simulink model "DCE_motor6_V2"  (R2025a)
settings: Solver=ode4  StartTime=0.0  StopTime=1  FixedStep=5e-5  RelTol=1e-3
undefined symbols (not defined in the file or in its folder): powergui
libraries: spsControlledVoltageSourceLib x24, spsControlledCurrentSourceLib x24, spsVoltageMeasurementLib x24, slpidlib x24, spspowerguiLib x2, simulink x1
(part 4 of 5)

== system DCE_motor6_V2/joint4/Motor2 ==
  TL : Inport
  IR_in : Inport  Port=2
  L_in : Inport  Port=3
  psi_in : Inport  Port=4
  2 : Gain  Gain=4
  Connector : Subsystem
  Constant : Constant  Value=-pi/2
  Constant1 : Constant  Value=2*pi
  Constant2 : Constant  Value=2*pi
  Gain : Gain  Gain=-50
  Integrator : Integrator
  Mechanical : Subsystem
  Mod : Math  Operator=mod
  Mod1 : Math  Operator=mod
  Mod2 : Math  Operator=mod
  Mux : Mux  Inputs=2
  P : Gain  Gain=50
  Product{,1..2,4} (4 alike) : Product
  Product3 : Product  Inputs=*/
  Sin : Trigonometry
  Sin1 : Trigonometry
  Sin2 : Trigonometry
  Sum : Sum  Inputs=+--
  Sum of Elements : Sum  Inputs=+
  Sum1 : Sum
  Sum2 : Sum
  Td : Gain  Gain=-0.003
  A+ : PMIOPort  Side=Left
  A- : PMIOPort  Port=2  Side=Left
  B+ : PMIOPort  Port=3  Side=Left
  B- : PMIOPort  Port=4  Side=Left
  Vp : Outport
  Ip : Outport  Port=2
  Te : Outport  Port=3
  w : Outport  Port=4
  theta : Outport  Port=5
  wires:
  Sum/1 -> Product3/1
  P/1 -> Mod1/1, 2/1, Sum2/1
  Mechanical/2(theta) -> theta/1, P/1
  Mechanical/1(w) -> Product1/2, w/1
  Product/1 -> Sum of Elements/1
  Sin2/1 -> Td/1
  Td/1 -> Sum1/2
  Sin1/1 -> Mux/1
  Integrator/1 -> Product2/1, Product/1, Ip/1, Connector/1(Ip)
  Constant/1 -> Sum2/2
  Sum of Elements/1 -> Sum1/1
  Connector/1(Vp) -> Vp/1, Sum/1
  Mux/1 -> Product4/1
  Sin/1 -> Mux/2
  Product1/1 -> Sum/2
  Sum1/1 -> Te/1, Mechanical/2(Te)
  TL/1 -> Mechanical/1(TL)
  Mod1/1 -> Sin1/1
  Mod/1 -> Sin/1
  Sum2/1 -> Mod/1
  Constant2/1 -> Mod/2
  Constant1/1 -> Mod1/2, Mod2/2
  Mod2/1 -> Sin2/1
  2/1 -> Mod2/1
  Product2/1 -> Sum/3
  IR_in/1 -> Product2/2
  Product3/1 -> Integrator/1
  L_in/1 -> Product3/2
  Product4/1 -> Product/2, Product1/1
  psi_in/1 -> Gain/1
  Gain/1 -> Product4/2
  connections:
  Connector/LConn4 -- B-/RConn1
  Connector/LConn3 -- B+/RConn1
  Connector/LConn2 -- A-/RConn1
  Connector/LConn1 -- A+/RConn1

== system DCE_motor6_V2/joint5/Mini08-1 ==
  In2 : Inport
  w : Inport  Port=2
  角度增益 : Gain  Gain=1/50
  转速增益 : Gain  Gain=1/50
  "Theta " : Outport
  "w " : Outport  Port=2
  wires:
  In2/1 -> 角度增益/1
  角度增益/1 -> "Theta "/1
  转速增益/1 -> "w "/1
  w/1 -> 转速增益/1

== system DCE_motor6_V2/joint5/Mini08-2 ==
  In2 : Inport
  w : Inport  Port=2
  角度增益 : Gain  Gain=1/50
  转速增益 : Gain  Gain=1/50
  "Theta " : Outport
  "w " : Outport  Port=2
  wires:
  In2/1 -> 角度增益/1
  角度增益/1 -> "Theta "/1
  转速增益/1 -> "w "/1
  w/1 -> 转速增益/1

== system DCE_motor6_V2/joint5/More Info2 ==

== system DCE_motor6_V2/joint5/Motor1 ==
  TL : Inport
  IR_in : Inport  Port=2
  L_in : Inport  Port=3
  psi_in : Inport  Port=4
  2 : Gain  Gain=4
  Connector : Subsystem
  Constant : Constant  Value=-pi/2
  Constant1 : Constant  Value=2*pi
  Constant2 : Constant  Value=2*pi
  Gain : Gain  Gain=-50
  Integrator : Integrator
  Mechanical : Subsystem
  Mod : Math  Operator=mod
  Mod1 : Math  Operator=mod
  Mod2 : Math  Operator=mod
  Mux : Mux  Inputs=2
  P : Gain  Gain=50
  Product{,1..2,4} (4 alike) : Product
  Product3 : Product  Inputs=*/
  Sin : Trigonometry
  Sin1 : Trigonometry
  Sin2 : Trigonometry
  Sum : Sum  Inputs=+--
  Sum of Elements : Sum  Inputs=+
  Sum1 : Sum
  Sum2 : Sum
  Td : Gain  Gain=-0.003
  A+ : PMIOPort  Side=Left
  A- : PMIOPort  Port=2  Side=Left
  B+ : PMIOPort  Port=3  Side=Left
  B- : PMIOPort  Port=4  Side=Left
  Vp : Outport
  Ip : Outport  Port=2
  Te : Outport  Port=3
  w : Outport  Port=4
  theta : Outport  Port=5
  wires:
  Sum/1 -> Product3/1
  P/1 -> Mod1/1, 2/1, Sum2/1
  Mechanical/2(theta) -> theta/1, P/1
  Mechanical/1(w) -> Product1/2, w/1
  Product/1 -> Sum of Elements/1
  Sin2/1 -> Td/1
  Td/1 -> Sum1/2
  Sin1/1 -> Mux/1
  Integrator/1 -> Product2/1, Product/1, Ip/1, Connector/1(Ip)
  Constant/1 -> Sum2/2
  Sum of Elements/1 -> Sum1/1
  Connector/1(Vp) -> Vp/1, Sum/1
  Mux/1 -> Product4/1
  Sin/1 -> Mux/2
  Product1/1 -> Sum/2
  Sum1/1 -> Te/1, Mechanical/2(Te)
  TL/1 -> Mechanical/1(TL)
  Mod1/1 -> Sin1/1
  Mod/1 -> Sin/1
  Sum2/1 -> Mod/1
  Constant2/1 -> Mod/2
  Constant1/1 -> Mod1/2, Mod2/2
  Mod2/1 -> Sin2/1
  2/1 -> Mod2/1
  Product2/1 -> Sum/3
  IR_in/1 -> Product2/2
  Product3/1 -> Integrator/1
  L_in/1 -> Product3/2
  Product4/1 -> Product/2, Product1/1
  psi_in/1 -> Gain/1
  Gain/1 -> Product4/2
  connections:
  Connector/LConn4 -- B-/RConn1
  Connector/LConn3 -- B+/RConn1
  Connector/LConn2 -- A-/RConn1
  Connector/LConn1 -- A+/RConn1

== system DCE_motor6_V2/joint5/Motor2 ==
  TL : Inport
  IR_in : Inport  Port=2
  L_in : Inport  Port=3
  psi_in : Inport  Port=4
  2 : Gain  Gain=4
  Connector : Subsystem
  Constant : Constant  Value=-pi/2
  Constant1 : Constant  Value=2*pi
  Constant2 : Constant  Value=2*pi
  Gain : Gain  Gain=-50
  Integrator : Integrator
  Mechanical : Subsystem
  Mod : Math  Operator=mod
  Mod1 : Math  Operator=mod
  Mod2 : Math  Operator=mod
  Mux : Mux  Inputs=2
  P : Gain  Gain=50
  Product{,1..2,4} (4 alike) : Product
  Product3 : Product  Inputs=*/
  Sin : Trigonometry
  Sin1 : Trigonometry
  Sin2 : Trigonometry
  Sum : Sum  Inputs=+--
  Sum of Elements : Sum  Inputs=+
  Sum1 : Sum
  Sum2 : Sum
  Td : Gain  Gain=-0.003
  A+ : PMIOPort  Side=Left
  A- : PMIOPort  Port=2  Side=Left
  B+ : PMIOPort  Port=3  Side=Left
  B- : PMIOPort  Port=4  Side=Left
  Vp : Outport
  Ip : Outport  Port=2
  Te : Outport  Port=3
  w : Outport  Port=4
  theta : Outport  Port=5
  wires:
  Sum/1 -> Product3/1
  P/1 -> Mod1/1, 2/1, Sum2/1
  Mechanical/2(theta) -> theta/1, P/1
  Mechanical/1(w) -> Product1/2, w/1
  Product/1 -> Sum of Elements/1
  Sin2/1 -> Td/1
  Td/1 -> Sum1/2
  Sin1/1 -> Mux/1
  Integrator/1 -> Product2/1, Product/1, Ip/1, Connector/1(Ip)
  Constant/1 -> Sum2/2
  Sum of Elements/1 -> Sum1/1
  Connector/1(Vp) -> Vp/1, Sum/1
  Mux/1 -> Product4/1
  Sin/1 -> Mux/2
  Product1/1 -> Sum/2
  Sum1/1 -> Te/1, Mechanical/2(Te)
  TL/1 -> Mechanical/1(TL)
  Mod1/1 -> Sin1/1
  Mod/1 -> Sin/1
  Sum2/1 -> Mod/1
  Constant2/1 -> Mod/2
  Constant1/1 -> Mod1/2, Mod2/2
  Mod2/1 -> Sin2/1
  2/1 -> Mod2/1
  Product2/1 -> Sum/3
  IR_in/1 -> Product2/2
  Product3/1 -> Integrator/1
  L_in/1 -> Product3/2
  Product4/1 -> Product/2, Product1/1
  psi_in/1 -> Gain/1
  Gain/1 -> Product4/2
  connections:
  Connector/LConn4 -- B-/RConn1
  Connector/LConn3 -- B+/RConn1
  Connector/LConn2 -- A-/RConn1
  Connector/LConn1 -- A+/RConn1

== system DCE_motor6_V2/joint6/Mini08-1 ==
  In2 : Inport
  w : Inport  Port=2
  角度增益 : Gain  Gain=1/50
  转速增益 : Gain  Gain=1/50
  "Theta " : Outport
  "w " : Outport  Port=2
  wires:
  In2/1 -> 角度增益/1
  角度增益/1 -> "Theta "/1
  转速增益/1 -> "w "/1
  w/1 -> 转速增益/1

== system DCE_motor6_V2/joint6/Mini08-2 ==
  In2 : Inport
  w : Inport  Port=2
  角度增益 : Gain  Gain=1/50
  转速增益 : Gain  Gain=1/50
  "Theta " : Outport
  "w " : Outport  Port=2
  wires:
  In2/1 -> 角度增益/1
  角度增益/1 -> "Theta "/1
  转速增益/1 -> "w "/1
  w/1 -> 转速增益/1

== system DCE_motor6_V2/joint6/Motor1 ==
  TL : Inport
  IR_in : Inport  Port=2
  L_in : Inport  Port=3
  psi_in : Inport  Port=4
  2 : Gain  Gain=4
  Connector : Subsystem
  Constant : Constant  Value=-pi/2
  Constant1 : Constant  Value=2*pi
  Constant2 : Constant  Value=2*pi
  Gain : Gain  Gain=-50
  Integrator : Integrator
  Mechanical : Subsystem
  Mod : Math  Operator=mod
  Mod1 : Math  Operator=mod
  Mod2 : Math  Operator=mod
  Mux : Mux  Inputs=2
  P : Gain  Gain=50
  Product{,1..2,4} (4 alike) : Product
  Product3 : Product  Inputs=*/
  Sin : Trigonometry
  Sin1 : Trigonometry
  Sin2 : Trigonometry
  Sum : Sum  Inputs=+--
  Sum of Elements : Sum  Inputs=+
  Sum1 : Sum
  Sum2 : Sum
  Td : Gain  Gain=-0.003
  A+ : PMIOPort  Side=Left
  A- : PMIOPort  Port=2  Side=Left
  B+ : PMIOPort  Port=3  Side=Left
  B- : PMIOPort  Port=4  Side=Left
  Vp : Outport
  Ip : Outport  Port=2
  Te : Outport  Port=3
  w : Outport  Port=4
  theta : Outport  Port=5
  wires:
  Sum/1 -> Product3/1
  P/1 -> Mod1/1, 2/1, Sum2/1
  Mechanical/2(theta) -> theta/1, P/1
  Mechanical/1(w) -> Product1/2, w/1
  Product/1 -> Sum of Elements/1
  Sin2/1 -> Td/1
  Td/1 -> Sum1/2
  Sin1/1 -> Mux/1
  Integrator/1 -> Product2/1, Product/1, Ip/1, Connector/1(Ip)
  Constant/1 -> Sum2/2
  Sum of Elements/1 -> Sum1/1
  Connector/1(Vp) -> Vp/1, Sum/1
  Mux/1 -> Product4/1
  Sin/1 -> Mux/2
  Product1/1 -> Sum/2
  Sum1/1 -> Te/1, Mechanical/2(Te)
  TL/1 -> Mechanical/1(TL)
  Mod1/1 -> Sin1/1
  Mod/1 -> Sin/1
  Sum2/1 -> Mod/1
  Constant2/1 -> Mod/2
  Constant1/1 -> Mod1/2, Mod2/2
  Mod2/1 -> Sin2/1
  2/1 -> Mod2/1
  Product2/1 -> Sum/3
  IR_in/1 -> Product2/2
  Product3/1 -> Integrator/1
  L_in/1 -> Product3/2
  Product4/1 -> Product/2, Product1/1
  psi_in/1 -> Gain/1
  Gain/1 -> Product4/2
  connections:
  Connector/LConn4 -- B-/RConn1
  Connector/LConn3 -- B+/RConn1
  Connector/LConn2 -- A-/RConn1
  Connector/LConn1 -- A+/RConn1

== system DCE_motor6_V2/joint6/Motor2 ==
  TL : Inport
  IR_in : Inport  Port=2
  L_in : Inport  Port=3
  psi_in : Inport  Port=4
  2 : Gain  Gain=4
  Connector : Subsystem
  Constant : Constant  Value=-pi/2
  Constant1 : Constant  Value=2*pi
  Constant2 : Constant  Value=2*pi
  Gain : Gain  Gain=-50
  Integrator : Integrator
  Mechanical : Subsystem
  Mod : Math  Operator=mod
  Mod1 : Math  Operator=mod
  Mod2 : Math  Operator=mod
  Mux : Mux  Inputs=2
  P : Gain  Gain=50
  Product{,1..2,4} (4 alike) : Product
  Product3 : Product  Inputs=*/
  Sin : Trigonometry
  Sin1 : Trigonometry
  Sin2 : Trigonometry
  Sum : Sum  Inputs=+--
  Sum of Elements : Sum  Inputs=+
  Sum1 : Sum
  Sum2 : Sum
  Td : Gain  Gain=-0.003
  A+ : PMIOPort  Side=Left
  A- : PMIOPort  Port=2  Side=Left
  B+ : PMIOPort  Port=3  Side=Left
  B- : PMIOPort  Port=4  Side=Left
  Vp : Outport
  Ip : Outport  Port=2
  Te : Outport  Port=3
  w : Outport  Port=4
  theta : Outport  Port=5
  wires:
  Sum/1 -> Product3/1
  P/1 -> Mod1/1, 2/1, Sum2/1
  Mechanical/2(theta) -> theta/1, P/1
  Mechanical/1(w) -> Product1/2, w/1
  Product/1 -> Sum of Elements/1
  Sin2/1 -> Td/1
  Td/1 -> Sum1/2
  Sin1/1 -> Mux/1
  Integrator/1 -> Product2/1, Product/1, Ip/1, Connector/1(Ip)
  Constant/1 -> Sum2/2
  Sum of Elements/1 -> Sum1/1
  Connector/1(Vp) -> Vp/1, Sum/1
  Mux/1 -> Product4/1
  Sin/1 -> Mux/2
  Product1/1 -> Sum/2
  Sum1/1 -> Te/1, Mechanical/2(Te)
  TL/1 -> Mechanical/1(TL)
  Mod1/1 -> Sin1/1
  Mod/1 -> Sin/1
  Sum2/1 -> Mod/1
  Constant2/1 -> Mod/2
  Constant1/1 -> Mod1/2, Mod2/2
  Mod2/1 -> Sin2/1
  2/1 -> Mod2/1
  Product2/1 -> Sum/3
  IR_in/1 -> Product2/2
  Product3/1 -> Integrator/1
  L_in/1 -> Product3/2
  Product4/1 -> Product/2, Product1/1
  psi_in/1 -> Gain/1
  Gain/1 -> Product4/2
  connections:
  Connector/LConn4 -- B-/RConn1
  Connector/LConn3 -- B+/RConn1
  Connector/LConn2 -- A-/RConn1
  Connector/LConn1 -- A+/RConn1

== system DCE_motor6_V2/powergui1/EquivalentModel1 ==
  Sources : Subsystem
  State-Space : S-Function  FunctionName=sfun_spssw_discc  Parameters=S.Ts,S.A, S.B, S.C, S.D, S.x0,S.EnableUseOfTLC  SFunctionDeploymentMode=off  EnableBusSupport=off
  Yout : Subsystem
  wires:
  State-Space/1 -> Yout/1(v,i)
  Sources/1(u) -> State-Space/1

== system DCE_motor6_V2/powergui1/EquivalentModel10 ==
  Sources : Subsystem
  State-Space : S-Function  FunctionName=sfun_spssw_discc  Parameters=S.Ts,S.A, S.B, S.C, S.D, S.x0,S.EnableUseOfTLC  SFunctionDeploymentMode=off  EnableBusSupport=off
  Yout : Subsystem
  wires:
  State-Space/1 -> Yout/1(v,i)
  Sources/1(u) -> State-Space/1

== system DCE_motor6_V2/powergui1/EquivalentModel11 ==
  Sources : Subsystem
  State-Space : S-Function  FunctionName=sfun_spssw_discc  Parameters=S.Ts,S.A, S.B, S.C, S.D, S.x0,S.EnableUseOfTLC  SFunctionDeploymentMode=off  EnableBusSupport=off
  Yout : Subsystem
  wires:
  State-Space/1 -> Yout/1(v,i)
  Sources/1(u) -> State-Space/1

== system DCE_motor6_V2/powergui1/EquivalentModel12 ==
  Sources : Subsystem
  State-Space : S-Function  FunctionName=sfun_spssw_discc  Parameters=S.Ts,S.A, S.B, S.C, S.D, S.x0,S.EnableUseOfTLC  SFunctionDeploymentMode=off  EnableBusSupport=off
  Yout : Subsystem
  wires:
  State-Space/1 -> Yout/1(v,i)
  Sources/1(u) -> State-Space/1

== system DCE_motor6_V2/powergui1/EquivalentModel13 ==
  Sources : Subsystem
  State-Space : S-Function  FunctionName=sfun_spssw_discc  Parameters=S.Ts,S.A, S.B, S.C, S.D, S.x0,S.EnableUseOfTLC  SFunctionDeploymentMode=off  EnableBusSupport=off
  Yout : Subsystem
  wires:
  State-Space/1 -> Yout/1(v,i)
  Sources/1(u) -> State-Space/1

== system DCE_motor6_V2/powergui1/EquivalentModel14 ==
  Sources : Subsystem
  State-Space : S-Function  FunctionName=sfun_spssw_discc  Parameters=S.Ts,S.A, S.B, S.C, S.D, S.x0,S.EnableUseOfTLC  SFunctionDeploymentMode=off  EnableBusSupport=off
  Yout : Subsystem
  wires:
  State-Space/1 -> Yout/1(v,i)
  Sources/1(u) -> State-Space/1

== system DCE_motor6_V2/powergui1/EquivalentModel15 ==
  Sources : Subsystem
  State-Space : S-Function  FunctionName=sfun_spssw_discc  Parameters=S.Ts,S.A, S.B, S.C, S.D, S.x0,S.EnableUseOfTLC  SFunctionDeploymentMode=off  EnableBusSupport=off
  Yout : Subsystem
  wires:
  State-Space/1 -> Yout/1(v,i)
  Sources/1(u) -> State-Space/1

== system DCE_motor6_V2/powergui1/EquivalentModel16 ==
  Sources : Subsystem
  State-Space : S-Function  FunctionName=sfun_spssw_discc  Parameters=S.Ts,S.A, S.B, S.C, S.D, S.x0,S.EnableUseOfTLC  SFunctionDeploymentMode=off  EnableBusSupport=off
  Yout : Subsystem
  wires:
  State-Space/1 -> Yout/1(v,i)
  Sources/1(u) -> State-Space/1

== system DCE_motor6_V2/powergui1/EquivalentModel17 ==
  Sources : Subsystem
  State-Space : S-Function  FunctionName=sfun_spssw_discc  Parameters=S.Ts,S.A, S.B, S.C, S.D, S.x0,S.EnableUseOfTLC  SFunctionDeploymentMode=off  EnableBusSupport=off
  Yout : Subsystem
  wires:
  State-Space/1 -> Yout/1(v,i)
  Sources/1(u) -> State-Space/1

== system DCE_motor6_V2/powergui1/EquivalentModel18 ==
  Sources : Subsystem
  State-Space : S-Function  FunctionName=sfun_spssw_discc  Parameters=S.Ts,S.A, S.B, S.C, S.D, S.x0,S.EnableUseOfTLC  SFunctionDeploymentMode=off  EnableBusSupport=off
  Yout : Subsystem
  wires:
  State-Space/1 -> Yout/1(v,i)
  Sources/1(u) -> State-Space/1

== system DCE_motor6_V2/powergui1/EquivalentModel19 ==
  Sources : Subsystem
  State-Space : S-Function  FunctionName=sfun_spssw_discc  Parameters=S.Ts,S.A, S.B, S.C, S.D, S.x0,S.EnableUseOfTLC  SFunctionDeploymentMode=off  EnableBusSupport=off
  Yout : Subsystem
  wires:
  State-Space/1 -> Yout/1(v,i)
  Sources/1(u) -> State-Space/1

== system DCE_motor6_V2/powergui1/EquivalentModel2 ==
  Sources : Subsystem
  State-Space : S-Function  FunctionName=sfun_spssw_discc  Parameters=S.Ts,S.A, S.B, S.C, S.D, S.x0,S.EnableUseOfTLC  SFunctionDeploymentMode=off  EnableBusSupport=off
  Yout : Subsystem
  wires:
  State-Space/1 -> Yout/1(v,i)
  Sources/1(u) -> State-Space/1

== system DCE_motor6_V2/powergui1/EquivalentModel20 ==
  Sources : Subsystem
  State-Space : S-Function  FunctionName=sfun_spssw_discc  Parameters=S.Ts,S.A, S.B, S.C, S.D, S.x0,S.EnableUseOfTLC  SFunctionDeploymentMode=off  EnableBusSupport=off
  Yout : Subsystem
  wires:
  State-Space/1 -> Yout/1(v,i)
  Sources/1(u) -> State-Space/1

== system DCE_motor6_V2/powergui1/EquivalentModel21 ==
  Sources : Subsystem
  State-Space : S-Function  FunctionName=sfun_spssw_discc  Parameters=S.Ts,S.A, S.B, S.C, S.D, S.x0,S.EnableUseOfTLC  SFunctionDeploymentMode=off  EnableBusSupport=off
  Yout : Subsystem
  wires:
  State-Space/1 -> Yout/1(v,i)
  Sources/1(u) -> State-Space/1

== system DCE_motor6_V2/powergui1/EquivalentModel22 ==
  Sources : Subsystem
  State-Space : S-Function  FunctionName=sfun_spssw_discc  Parameters=S.Ts,S.A, S.B, S.C, S.D, S.x0,S.EnableUseOfTLC  SFunctionDeploymentMode=off  EnableBusSupport=off
  Yout : Subsystem
  wires:
  State-Space/1 -> Yout/1(v,i)
  Sources/1(u) -> State-Space/1

== system DCE_motor6_V2/powergui1/EquivalentModel23 ==
  Sources : Subsystem
  State-Space : S-Function  FunctionName=sfun_spssw_discc  Parameters=S.Ts,S.A, S.B, S.C, S.D, S.x0,S.EnableUseOfTLC  SFunctionDeploymentMode=off  EnableBusSupport=off
  Yout : Subsystem
  wires:
  State-Space/1 -> Yout/1(v,i)
  Sources/1(u) -> State-Space/1

== system DCE_motor6_V2/powergui1/EquivalentModel24 ==
  Sources : Subsystem
  State-Space : S-Function  FunctionName=sfun_spssw_discc  Parameters=S.Ts,S.A, S.B, S.C, S.D, S.x0,S.EnableUseOfTLC  SFunctionDeploymentMode=off  EnableBusSupport=off
  Yout : Subsystem
  wires:
  State-Space/1 -> Yout/1(v,i)
  Sources/1(u) -> State-Space/1

== system DCE_motor6_V2/powergui1/EquivalentModel3 ==
  Sources : Subsystem
  State-Space : S-Function  FunctionName=sfun_spssw_discc  Parameters=S.Ts,S.A, S.B, S.C, S.D, S.x0,S.EnableUseOfTLC  SFunctionDeploymentMode=off  EnableBusSupport=off
  Yout : Subsystem
  wires:
  State-Space/1 -> Yout/1(v,i)
  Sources/1(u) -> State-Space/1

== system DCE_motor6_V2/powergui1/EquivalentModel4 ==
  Sources : Subsystem
  State-Space : S-Function  FunctionName=sfun_spssw_discc  Parameters=S.Ts,S.A, S.B, S.C, S.D, S.x0,S.EnableUseOfTLC  SFunctionDeploymentMode=off  EnableBusSupport=off
  Yout : Subsystem
  wires:
  State-Space/1 -> Yout/1(v,i)
  Sources/1(u) -> State-Space/1

== system DCE_motor6_V2/powergui1/EquivalentModel5 ==
  Sources : Subsystem
  State-Space : S-Function  FunctionName=sfun_spssw_discc  Parameters=S.Ts,S.A, S.B, S.C, S.D, S.x0,S.EnableUseOfTLC  SFunctionDeploymentMode=off  EnableBusSupport=off
  Yout : Subsystem
  wires:
  State-Space/1 -> Yout/1(v,i)
  Sources/1(u) -> State-Space/1

== system DCE_motor6_V2/powergui1/EquivalentModel6 ==
  Sources : Subsystem
  State-Space : S-Function  FunctionName=sfun_spssw_discc  Parameters=S.Ts,S.A, S.B, S.C, S.D, S.x0,S.EnableUseOfTLC  SFunctionDeploymentMode=off  EnableBusSupport=off
  Yout : Subsystem
  wires:
  State-Space/1 -> Yout/1(v,i)
  Sources/1(u) -> State-Space/1

== system DCE_motor6_V2/powergui1/EquivalentModel7 ==
  Sources : Subsystem
  State-Space : S-Function  FunctionName=sfun_spssw_discc  Parameters=S.Ts,S.A, S.B, S.C, S.D, S.x0,S.EnableUseOfTLC  SFunctionDeploymentMode=off  EnableBusSupport=off
  Yout : Subsystem
  wires:
  State-Space/1 -> Yout/1(v,i)
  Sources/1(u) -> State-Space/1

== system DCE_motor6_V2/powergui1/EquivalentModel8 ==
  Sources : Subsystem
  State-Space : S-Function  FunctionName=sfun_spssw_discc  Parameters=S.Ts,S.A, S.B, S.C, S.D, S.x0,S.EnableUseOfTLC  SFunctionDeploymentMode=off  EnableBusSupport=off
  Yout : Subsystem
  wires:
  State-Space/1 -> Yout/1(v,i)
  Sources/1(u) -> State-Space/1

== system DCE_motor6_V2/powergui1/EquivalentModel9 ==
  Sources : Subsystem
  State-Space : S-Function  FunctionName=sfun_spssw_discc  Parameters=S.Ts,S.A, S.B, S.C, S.D, S.x0,S.EnableUseOfTLC  SFunctionDeploymentMode=off  EnableBusSupport=off
  Yout : Subsystem
  wires:
  State-Space/1 -> Yout/1(v,i)
  Sources/1(u) -> State-Space/1

== system DCE_motor6_V2/joint1/Motor1/Connector ==
  Ip : Inport
  Controlled Current Source : spsControlledCurrentSourceLib/Controlled Current Source  Initialize=on  Source_Type=AC  Amplitude=2  Phase=0  Frequency=0  Measurements=None
  Controlled Current Source1 : spsControlledCurrentSourceLib/Controlled Current Source  Initialize=on  Source_Type=AC  Amplitude=2  Phase=0  Frequency=0  Measurements=None
  Demux : Demux  Outputs=2
  Mux : Mux  Inputs=2
  Scope6 : Scope  NumInputPorts=2
      settings: ActiveDisplayYMinimum=-2.39364466431234  ActiveDisplayYMaximum=2.3993658884477673  DataLoggingVariableName=ScopeData5
  Voltage Measurement : spsVoltageMeasurementLib/Voltage Measurement  PhasorSimulation=off  OutputType=Complex  PSBequivalent=0
  Voltage Measurement1 : spsVoltageMeasurementLib/Voltage Measurement  PhasorSimulation=off  OutputType=Complex  PSBequivalent=0
  A+ : PMIOPort  Side=Left
  A- : PMIOPort  Port=2  Side=Left
  B+ : PMIOPort  Port=3  Side=Left
  B- : PMIOPort  Port=4  Side=Left
  Vp : Outport
  wires:
  Mux/1 -> Vp/1
  Ip/1 -> Demux/1
  Demux/1 -> Controlled Current Source/1
  Demux/2 -> Controlled Current Source1/1
  Voltage Measurement/1 -> Scope6/1, Mux/1  "Va"
  Voltage Measurement1/1 -> Scope6/2, Mux/2  "Vb"
  connections:
  A+/RConn1 -- Controlled Current Source/LConn1 -- Voltage Measurement/LConn1
  A-/RConn1 -- Controlled Current Source/RConn1 -- Voltage Measurement/LConn2
  B+/RConn1 -- Voltage Measurement1/LConn1 -- Controlled Current Source1/LConn1
  B-/RConn1 -- Controlled Current Source1/RConn1 -- Voltage Measurement1/LConn2

== system DCE_motor6_V2/joint1/Motor1/Mechanical ==
  TL : Inport
  Te : Inport  Port=2
  1/J : Gain  Gain=1/(1e-5)
  B : Gain  Gain=1e-4
  Integrator : Integrator
  Integrator1 : Integrator
  Sum : Sum  Inputs=-+-
  w : Outport
  theta : Outport  Port=2
  wires:
  Te/1 -> Sum/2
  TL/1 -> Sum/1
  Sum/1 -> 1/J/1
  1/J/1 -> Integrator/1
  Integrator/1 -> B/1, w/1, Integrator1/1  "w"
  Integrator1/1 -> theta/1  "theta"
  B/1 -> Sum/3

== system DCE_motor6_V2/joint1/Motor2/Connector ==
  Ip : Inport
  Controlled Current Source : spsControlledCurrentSourceLib/Controlled Current Source  Initialize=on  Source_Type=AC  Amplitude=2  Phase=0  Frequency=0  Measurements=None
  Controlled Current Source1 : spsControlledCurrentSourceLib/Controlled Current Source  Initialize=on  Source_Type=AC  Amplitude=2  Phase=0  Frequency=0  Measurements=None
  Demux : Demux  Outputs=2
  Mux : Mux  Inputs=2
  Scope6 : Scope  NumInputPorts=2
      settings: ActiveDisplayYMinimum=-2.39364466431234  ActiveDisplayYMaximum=2.3993658884477673  DataLoggingVariableName=ScopeData5
  Voltage Measurement : spsVoltageMeasurementLib/Voltage Measurement  PhasorSimulation=off  OutputType=Complex  PSBequivalent=0
  Voltage Measurement1 : spsVoltageMeasurementLib/Voltage Measurement  PhasorSimulation=off  OutputType=Complex  PSBequivalent=0
  A+ : PMIOPort  Side=Left
  A- : PMIOPort  Port=2  Side=Left
  B+ : PMIOPort  Port=3  Side=Left
  B- : PMIOPort  Port=4  Side=Left
  Vp : Outport
  wires:
  Mux/1 -> Vp/1
  Ip/1 -> Demux/1
  Demux/1 -> Controlled Current Source/1
  Demux/2 -> Controlled Current Source1/1
  Voltage Measurement/1 -> Scope6/1, Mux/1  "Va"
  Voltage Measurement1/1 -> Scope6/2, Mux/2  "Vb"
  connections:
  A+/RConn1 -- Controlled Current Source/LConn1 -- Voltage Measurement/LConn1
  A-/RConn1 -- Controlled Current Source/RConn1 -- Voltage Measurement/LConn2
  B+/RConn1 -- Voltage Measurement1/LConn1 -- Controlled Current Source1/LConn1
  B-/RConn1 -- Controlled Current Source1/RConn1 -- Voltage Measurement1/LConn2

== system DCE_motor6_V2/joint1/Motor2/Mechanical ==
  TL : Inport
  Te : Inport  Port=2
  1/J : Gain  Gain=1/(1e-5)
  B : Gain  Gain=1e-4
  Integrator : Integrator
  Integrator1 : Integrator
  Sum : Sum  Inputs=-+-
  w : Outport
  theta : Outport  Port=2
  wires:
  Te/1 -> Sum/2
  TL/1 -> Sum/1
  Sum/1 -> 1/J/1
  1/J/1 -> Integrator/1
  Integrator/1 -> B/1, w/1, Integrator1/1  "w"
  Integrator1/1 -> theta/1  "theta"
  B/1 -> Sum/3

== system DCE_motor6_V2/joint2/Motor1/Connector ==
  Ip : Inport
  Controlled Current Source : spsControlledCurrentSourceLib/Controlled Current Source  Initialize=on  Source_Type=AC  Amplitude=2  Phase=0  Frequency=0  Measurements=None
  Controlled Current Source1 : spsControlledCurrentSourceLib/Controlled Current Source  Initialize=on  Source_Type=AC  Amplitude=2  Phase=0  Frequency=0  Measurements=None
  Demux : Demux  Outputs=2
  Mux : Mux  Inputs=2
  Scope6 : Scope  NumInputPorts=2
      settings: ActiveDisplayYMinimum=-2.39364466431234  ActiveDisplayYMaximum=2.3993658884477673  DataLoggingVariableName=ScopeData5
  Voltage Measurement : spsVoltageMeasurementLib/Voltage Measurement  PhasorSimulation=off  OutputType=Complex  PSBequivalent=0
  Voltage Measurement1 : spsVoltageMeasurementLib/Voltage Measurement  PhasorSimulation=off  OutputType=Complex  PSBequivalent=0
  A+ : PMIOPort  Side=Left
  A- : PMIOPort  Port=2  Side=Left
  B+ : PMIOPort  Port=3  Side=Left
  B- : PMIOPort  Port=4  Side=Left
  Vp : Outport
  wires:
  Mux/1 -> Vp/1
  Ip/1 -> Demux/1
  Demux/1 -> Controlled Current Source/1
  Demux/2 -> Controlled Current Source1/1
  Voltage Measurement/1 -> Scope6/1, Mux/1  "Va"
  Voltage Measurement1/1 -> Scope6/2, Mux/2  "Vb"
  connections:
  A+/RConn1 -- Controlled Current Source/LConn1 -- Voltage Measurement/LConn1
  A-/RConn1 -- Controlled Current Source/RConn1 -- Voltage Measurement/LConn2
  B+/RConn1 -- Voltage Measurement1/LConn1 -- Controlled Current Source1/LConn1
  B-/RConn1 -- Controlled Current Source1/RConn1 -- Voltage Measurement1/LConn2

== system DCE_motor6_V2/joint2/Motor1/Mechanical ==
  TL : Inport
  Te : Inport  Port=2
  1/J : Gain  Gain=1/(1e-5)
  B : Gain  Gain=1e-4
  Integrator : Integrator
  Integrator1 : Integrator
  Sum : Sum  Inputs=-+-
  w : Outport
  theta : Outport  Port=2
  wires:
  Te/1 -> Sum/2
  TL/1 -> Sum/1
  Sum/1 -> 1/J/1
  1/J/1 -> Integrator/1
  Integrator/1 -> B/1, w/1, Integrator1/1  "w"
  Integrator1/1 -> theta/1  "theta"
  B/1 -> Sum/3

== system DCE_motor6_V2/joint2/Motor2/Connector ==
  Ip : Inport
  Controlled Current Source : spsControlledCurrentSourceLib/Controlled Current Source  Initialize=on  Source_Type=AC  Amplitude=2  Phase=0  Frequency=0  Measurements=None
  Controlled Current Source1 : spsControlledCurrentSourceLib/Controlled Current Source  Initialize=on  Source_Type=AC  Amplitude=2  Phase=0  Frequency=0  Measurements=None
  Demux : Demux  Outputs=2
  Mux : Mux  Inputs=2
  Scope6 : Scope  NumInputPorts=2
      settings: ActiveDisplayYMinimum=-2.39364466431234  ActiveDisplayYMaximum=2.3993658884477673  DataLoggingVariableName=ScopeData5
  Voltage Measurement : spsVoltageMeasurementLib/Voltage Measurement  PhasorSimulation=off  OutputType=Complex  PSBequivalent=0
  Voltage Measurement1 : spsVoltageMeasurementLib/Voltage Measurement  PhasorSimulation=off  OutputType=Complex  PSBequivalent=0
  A+ : PMIOPort  Side=Left
  A- : PMIOPort  Port=2  Side=Left
  B+ : PMIOPort  Port=3  Side=Left
  B- : PMIOPort  Port=4  Side=Left
  Vp : Outport
  wires:
  Mux/1 -> Vp/1
  Ip/1 -> Demux/1
  Demux/1 -> Controlled Current Source/1
  Demux/2 -> Controlled Current Source1/1
  Voltage Measurement/1 -> Scope6/1, Mux/1  "Va"
  Voltage Measurement1/1 -> Scope6/2, Mux/2  "Vb"
  connections:
  A+/RConn1 -- Controlled Current Source/LConn1 -- Voltage Measurement/LConn1
  A-/RConn1 -- Controlled Current Source/RConn1 -- Voltage Measurement/LConn2
  B+/RConn1 -- Voltage Measurement1/LConn1 -- Controlled Current Source1/LConn1
  B-/RConn1 -- Controlled Current Source1/RConn1 -- Voltage Measurement1/LConn2

== system DCE_motor6_V2/joint2/Motor2/Mechanical ==
  TL : Inport
  Te : Inport  Port=2
  1/J : Gain  Gain=1/(1e-5)
  B : Gain  Gain=1e-4
  Integrator : Integrator
  Integrator1 : Integrator
  Sum : Sum  Inputs=-+-
  w : Outport
  theta : Outport  Port=2
  wires:
  Te/1 -> Sum/2
  TL/1 -> Sum/1
  Sum/1 -> 1/J/1
  1/J/1 -> Integrator/1
  Integrator/1 -> B/1, w/1, Integrator1/1  "w"
  Integrator1/1 -> theta/1  "theta"
  B/1 -> Sum/3

== system DCE_motor6_V2/joint3/Motor1/Connector ==
  Ip : Inport
  Controlled Current Source : spsControlledCurrentSourceLib/Controlled Current Source  Initialize=on  Source_Type=AC  Amplitude=2  Phase=0  Frequency=0  Measurements=None
  Controlled Current Source1 : spsControlledCurrentSourceLib/Controlled Current Source  Initialize=on  Source_Type=AC  Amplitude=2  Phase=0  Frequency=0  Measurements=None
  Demux : Demux  Outputs=2
  Mux : Mux  Inputs=2
  Scope6 : Scope  NumInputPorts=2
      settings: ActiveDisplayYMinimum=-2.39364466431234  ActiveDisplayYMaximum=2.3993658884477673  DataLoggingVariableName=ScopeData5
  Voltage Measurement : spsVoltageMeasurementLib/Voltage Measurement  PhasorSimulation=off  OutputType=Complex  PSBequivalent=0
  Voltage Measurement1 : spsVoltageMeasurementLib/Voltage Measurement  PhasorSimulation=off  OutputType=Complex  PSBequivalent=0
  A+ : PMIOPort  Side=Left
  A- : PMIOPort  Port=2  Side=Left
  B+ : PMIOPort  Port=3  Side=Left
  B- : PMIOPort  Port=4  Side=Left
  Vp : Outport
  wires:
  Mux/1 -> Vp/1
  Ip/1 -> Demux/1
  Demux/1 -> Controlled Current Source/1
  Demux/2 -> Controlled Current Source1/1
  Voltage Measurement/1 -> Scope6/1, Mux/1  "Va"
  Voltage Measurement1/1 -> Scope6/2, Mux/2  "Vb"
  connections:
  A+/RConn1 -- Controlled Current Source/LConn1 -- Voltage Measurement/LConn1
  A-/RConn1 -- Controlled Current Source/RConn1 -- Voltage Measurement/LConn2
  B+/RConn1 -- Voltage Measurement1/LConn1 -- Controlled Current Source1/LConn1
  B-/RConn1 -- Controlled Current Source1/RConn1 -- Voltage Measurement1/LConn2

== system DCE_motor6_V2/joint3/Motor1/Mechanical ==
  TL : Inport
  Te : Inport  Port=2
  1/J : Gain  Gain=1/(1e-5)
  B : Gain  Gain=1e-4
  Integrator : Integrator
  Integrator1 : Integrator
  Sum : Sum  Inputs=-+-
  w : Outport
  theta : Outport  Port=2
  wires:
  Te/1 -> Sum/2
  TL/1 -> Sum/1
  Sum/1 -> 1/J/1
  1/J/1 -> Integrator/1
  Integrator/1 -> B/1, w/1, Integrator1/1  "w"
  Integrator1/1 -> theta/1  "theta"
  B/1 -> Sum/3

== system DCE_motor6_V2/joint3/Motor2/Connector ==
  Ip : Inport
  Controlled Current Source : spsControlledCurrentSourceLib/Controlled Current Source  Initialize=on  Source_Type=AC  Amplitude=2  Phase=0  Frequency=0  Measurements=None
  Controlled Current Source1 : spsControlledCurrentSourceLib/Controlled Current Source  Initialize=on  Source_Type=AC  Amplitude=2  Phase=0  Frequency=0  Measurements=None
  Demux : Demux  Outputs=2
  Mux : Mux  Inputs=2
  Scope6 : Scope  NumInputPorts=2
      settings: ActiveDisplayYMinimum=-2.39364466431234  ActiveDisplayYMaximum=2.3993658884477673  DataLoggingVariableName=ScopeData5
  Voltage Measurement : spsVoltageMeasurementLib/Voltage Measurement  PhasorSimulation=off  OutputType=Complex  PSBequivalent=0
  Voltage Measurement1 : spsVoltageMeasurementLib/Voltage Measurement  PhasorSimulation=off  OutputType=Complex  PSBequivalent=0
  A+ : PMIOPort  Side=Left
  A- : PMIOPort  Port=2  Side=Left
  B+ : PMIOPort  Port=3  Side=Left
  B- : PMIOPort  Port=4  Side=Left
  Vp : Outport
  wires:
  Mux/1 -> Vp/1
  Ip/1 -> Demux/1
  Demux/1 -> Controlled Current Source/1
  Demux/2 -> Controlled Current Source1/1
  Voltage Measurement/1 -> Scope6/1, Mux/1  "Va"
  Voltage Measurement1/1 -> Scope6/2, Mux/2  "Vb"
  connections:
  A+/RConn1 -- Controlled Current Source/LConn1 -- Voltage Measurement/LConn1
  A-/RConn1 -- Controlled Current Source/RConn1 -- Voltage Measurement/LConn2
  B+/RConn1 -- Voltage Measurement1/LConn1 -- Controlled Current Source1/LConn1
  B-/RConn1 -- Controlled Current Source1/RConn1 -- Voltage Measurement1/LConn2

== system DCE_motor6_V2/joint3/Motor2/Mechanical ==
  TL : Inport
  Te : Inport  Port=2
  1/J : Gain  Gain=1/(1e-5)
  B : Gain  Gain=1e-4
  Integrator : Integrator
  Integrator1 : Integrator
  Sum : Sum  Inputs=-+-
  w : Outport
  theta : Outport  Port=2
  wires:
  Te/1 -> Sum/2
  TL/1 -> Sum/1
  Sum/1 -> 1/J/1
  1/J/1 -> Integrator/1
  Integrator/1 -> B/1, w/1, Integrator1/1  "w"
  Integrator1/1 -> theta/1  "theta"
  B/1 -> Sum/3

== system DCE_motor6_V2/joint4/Motor1/Connector ==
  Ip : Inport
  Controlled Current Source : spsControlledCurrentSourceLib/Controlled Current Source  Initialize=on  Source_Type=AC  Amplitude=2  Phase=0  Frequency=0  Measurements=None
  Controlled Current Source1 : spsControlledCurrentSourceLib/Controlled Current Source  Initialize=on  Source_Type=AC  Amplitude=2  Phase=0  Frequency=0  Measurements=None
  Demux : Demux  Outputs=2
  Mux : Mux  Inputs=2
  Scope6 : Scope  NumInputPorts=2
      settings: ActiveDisplayYMinimum=-2.39364466431234  ActiveDisplayYMaximum=2.3993658884477673  DataLoggingVariableName=ScopeData5
  Voltage Measurement : spsVoltageMeasurementLib/Voltage Measurement  PhasorSimulation=off  OutputType=Complex  PSBequivalent=0
  Voltage Measurement1 : spsVoltageMeasurementLib/Voltage Measurement  PhasorSimulation=off  OutputType=Complex  PSBequivalent=0
  A+ : PMIOPort  Side=Left
  A- : PMIOPort  Port=2  Side=Left
  B+ : PMIOPort  Port=3  Side=Left
  B- : PMIOPort  Port=4  Side=Left
  Vp : Outport
  wires:
  Mux/1 -> Vp/1
  Ip/1 -> Demux/1
  Demux/1 -> Controlled Current Source/1
  Demux/2 -> Controlled Current Source1/1
  Voltage Measurement/1 -> Scope6/1, Mux/1  "Va"
  Voltage Measurement1/1 -> Scope6/2, Mux/2  "Vb"
  connections:
  A+/RConn1 -- Controlled Current Source/LConn1 -- Voltage Measurement/LConn1
  A-/RConn1 -- Controlled Current Source/RConn1 -- Voltage Measurement/LConn2
  B+/RConn1 -- Voltage Measurement1/LConn1 -- Controlled Current Source1/LConn1
  B-/RConn1 -- Controlled Current Source1/RConn1 -- Voltage Measurement1/LConn2

== system DCE_motor6_V2/joint4/Motor1/Mechanical ==
  TL : Inport
  Te : Inport  Port=2
  1/J : Gain  Gain=1/(1e-5)
  B : Gain  Gain=1e-4
  Integrator : Integrator
  Integrator1 : Integrator
  Sum : Sum  Inputs=-+-
  w : Outport
  theta : Outport  Port=2
  wires:
  Te/1 -> Sum/2
  TL/1 -> Sum/1
  Sum/1 -> 1/J/1
  1/J/1 -> Integrator/1
  Integrator/1 -> B/1, w/1, Integrator1/1  "w"
  Integrator1/1 -> theta/1  "theta"
  B/1 -> Sum/3

== system DCE_motor6_V2/joint4/Motor2/Connector ==
  Ip : Inport
  Controlled Current Source : spsControlledCurrentSourceLib/Controlled Current Source  Initialize=on  Source_Type=AC  Amplitude=2  Phase=0  Frequency=0  Measurements=None
  Controlled Current Source1 : spsControlledCurrentSourceLib/Controlled Current Source  Initialize=on  Source_Type=AC  Amplitude=2  Phase=0  Frequency=0  Measurements=None
  Demux : Demux  Outputs=2
  Mux : Mux  Inputs=2
  Scope6 : Scope  NumInputPorts=2
      settings: ActiveDisplayYMinimum=-2.39364466431234  ActiveDisplayYMaximum=2.3993658884477673  DataLoggingVariableName=ScopeData5
  Voltage Measurement : spsVoltageMeasurementLib/Voltage Measurement  PhasorSimulation=off  OutputType=Complex  PSBequivalent=0
  Voltage Measurement1 : spsVoltageMeasurementLib/Voltage Measurement  PhasorSimulation=off  OutputType=Complex  PSBequivalent=0
  A+ : PMIOPort  Side=Left
  A- : PMIOPort  Port=2  Side=Left
  B+ : PMIOPort  Port=3  Side=Left
  B- : PMIOPort  Port=4  Side=Left
  Vp : Outport
  wires:
  Mux/1 -> Vp/1
  Ip/1 -> Demux/1
  Demux/1 -> Controlled Current Source/1
  Demux/2 -> Controlled Current Source1/1
  Voltage Measurement/1 -> Scope6/1, Mux/1  "Va"
  Voltage Measurement1/1 -> Scope6/2, Mux/2  "Vb"
  connections:
  A+/RConn1 -- Controlled Current Source/LConn1 -- Voltage Measurement/LConn1
  A-/RConn1 -- Controlled Current Source/RConn1 -- Voltage Measurement/LConn2
  B+/RConn1 -- Voltage Measurement1/LConn1 -- Controlled Current Source1/LConn1
  B-/RConn1 -- Controlled Current Source1/RConn1 -- Voltage Measurement1/LConn2

== system DCE_motor6_V2/joint4/Motor2/Mechanical ==
  TL : Inport
  Te : Inport  Port=2
  1/J : Gain  Gain=1/(1e-5)
  B : Gain  Gain=1e-4
  Integrator : Integrator
  Integrator1 : Integrator
  Sum : Sum  Inputs=-+-
  w : Outport
  theta : Outport  Port=2
  wires:
  Te/1 -> Sum/2
  TL/1 -> Sum/1
  Sum/1 -> 1/J/1
  1/J/1 -> Integrator/1
  Integrator/1 -> B/1, w/1, Integrator1/1  "w"
  Integrator1/1 -> theta/1  "theta"
  B/1 -> Sum/3

== system DCE_motor6_V2/joint5/Motor1/Connector ==
  Ip : Inport
  Controlled Current Source : spsControlledCurrentSourceLib/Controlled Current Source  Initialize=on  Source_Type=AC  Amplitude=2  Phase=0  Frequency=0  Measurements=None
  Controlled Current Source1 : spsControlledCurrentSourceLib/Controlled Current Source  Initialize=on  Source_Type=AC  Amplitude=2  Phase=0  Frequency=0  Measurements=None
  Demux : Demux  Outputs=2
  Mux : Mux  Inputs=2
  Scope6 : Scope  NumInputPorts=2
      settings: ActiveDisplayYMinimum=-2.39364466431234  ActiveDisplayYMaximum=2.3993658884477673  DataLoggingVariableName=ScopeData5
  Voltage Measurement : spsVoltageMeasurementLib/Voltage Measurement  PhasorSimulation=off  OutputType=Complex  PSBequivalent=0
  Voltage Measurement1 : spsVoltageMeasurementLib/Voltage Measurement  PhasorSimulation=off  OutputType=Complex  PSBequivalent=0
  A+ : PMIOPort  Side=Left
  A- : PMIOPort  Port=2  Side=Left
  B+ : PMIOPort  Port=3  Side=Left
  B- : PMIOPort  Port=4  Side=Left
  Vp : Outport
  wires:
  Mux/1 -> Vp/1
  Ip/1 -> Demux/1
  Demux/1 -> Controlled Current Source/1
  Demux/2 -> Controlled Current Source1/1
  Voltage Measurement/1 -> Scope6/1, Mux/1  "Va"
  Voltage Measurement1/1 -> Scope6/2, Mux/2  "Vb"
  connections:
  A+/RConn1 -- Controlled Current Source/LConn1 -- Voltage Measurement/LConn1
  A-/RConn1 -- Controlled Current Source/RConn1 -- Voltage Measurement/LConn2
  B+/RConn1 -- Voltage Measurement1/LConn1 -- Controlled Current Source1/LConn1
  B-/RConn1 -- Controlled Current Source1/RConn1 -- Voltage Measurement1/LConn2

== system DCE_motor6_V2/joint5/Motor1/Mechanical ==
  TL : Inport
  Te : Inport  Port=2
  1/J : Gain  Gain=1/(1e-5)
  B : Gain  Gain=1e-4
  Integrator : Integrator
  Integrator1 : Integrator
  Sum : Sum  Inputs=-+-
  w : Outport
  theta : Outport  Port=2
  wires:
  Te/1 -> Sum/2
  TL/1 -> Sum/1
  Sum/1 -> 1/J/1
  1/J/1 -> Integrator/1
  Integrator/1 -> B/1, w/1, Integrator1/1  "w"
  Integrator1/1 -> theta/1  "theta"
  B/1 -> Sum/3

== system DCE_motor6_V2/joint5/Motor2/Connector ==
  Ip : Inport
  Controlled Current Source : spsControlledCurrentSourceLib/Controlled Current Source  Initialize=on  Source_Type=AC  Amplitude=2  Phase=0  Frequency=0  Measurements=None
  Controlled Current Source1 : spsControlledCurrentSourceLib/Controlled Current Source  Initialize=on  Source_Type=AC  Amplitude=2  Phase=0  Frequency=0  Measurements=None
  Demux : Demux  Outputs=2
  Mux : Mux  Inputs=2
  Scope6 : Scope  NumInputPorts=2
      settings: ActiveDisplayYMinimum=-2.39364466431234  ActiveDisplayYMaximum=2.3993658884477673  DataLoggingVariableName=ScopeData5
  Voltage Measurement : spsVoltageMeasurementLib/Voltage Measurement  PhasorSimulation=off  OutputType=Complex  PSBequivalent=0
  Voltage Measurement1 : spsVoltageMeasurementLib/Voltage Measurement  PhasorSimulation=off  OutputType=Complex  PSBequivalent=0
  A+ : PMIOPort  Side=Left
  A- : PMIOPort  Port=2  Side=Left
  B+ : PMIOPort  Port=3  Side=Left
  B- : PMIOPort  Port=4  Side=Left
  Vp : Outport
  wires:
  Mux/1 -> Vp/1
  Ip/1 -> Demux/1
  Demux/1 -> Controlled Current Source/1
  Demux/2 -> Controlled Current Source1/1
  Voltage Measurement/1 -> Scope6/1, Mux/1  "Va"
  Voltage Measurement1/1 -> Scope6/2, Mux/2  "Vb"
  connections:
  A+/RConn1 -- Controlled Current Source/LConn1 -- Voltage Measurement/LConn1
  A-/RConn1 -- Controlled Current Source/RConn1 -- Voltage Measurement/LConn2
  B+/RConn1 -- Voltage Measurement1/LConn1 -- Controlled Current Source1/LConn1
  B-/RConn1 -- Controlled Current Source1/RConn1 -- Voltage Measurement1/LConn2

== system DCE_motor6_V2/joint5/Motor2/Mechanical ==
  TL : Inport
  Te : Inport  Port=2
  1/J : Gain  Gain=1/(1e-5)
  B : Gain  Gain=1e-4
  Integrator : Integrator
  Integrator1 : Integrator
  Sum : Sum  Inputs=-+-
  w : Outport
  theta : Outport  Port=2
  wires:
  Te/1 -> Sum/2
  TL/1 -> Sum/1
  Sum/1 -> 1/J/1
  1/J/1 -> Integrator/1
  Integrator/1 -> B/1, w/1, Integrator1/1  "w"
  Integrator1/1 -> theta/1  "theta"
  B/1 -> Sum/3

== system DCE_motor6_V2/joint6/Motor1/Connector ==
  Ip : Inport
  Controlled Current Source : spsControlledCurrentSourceLib/Controlled Current Source  Initialize=on  Source_Type=AC  Amplitude=2  Phase=0  Frequency=0  Measurements=None
  Controlled Current Source1 : spsControlledCurrentSourceLib/Controlled Current Source  Initialize=on  Source_Type=AC  Amplitude=2  Phase=0  Frequency=0  Measurements=None
  Demux : Demux  Outputs=2
  Mux : Mux  Inputs=2
  Scope6 : Scope  NumInputPorts=2
      settings: ActiveDisplayYMinimum=-2.39364466431234  ActiveDisplayYMaximum=2.3993658884477673  DataLoggingVariableName=ScopeData5
  Voltage Measurement : spsVoltageMeasurementLib/Voltage Measurement  PhasorSimulation=off  OutputType=Complex  PSBequivalent=0
  Voltage Measurement1 : spsVoltageMeasurementLib/Voltage Measurement  PhasorSimulation=off  OutputType=Complex  PSBequivalent=0
  A+ : PMIOPort  Side=Left
  A- : PMIOPort  Port=2  Side=Left
  B+ : PMIOPort  Port=3  Side=Left
  B- : PMIOPort  Port=4  Side=Left
  Vp : Outport
  wires:
  Mux/1 -> Vp/1
  Ip/1 -> Demux/1
  Demux/1 -> Controlled Current Source/1
  Demux/2 -> Controlled Current Source1/1
  Voltage Measurement/1 -> Scope6/1, Mux/1  "Va"
  Voltage Measurement1/1 -> Scope6/2, Mux/2  "Vb"
  connections:
  A+/RConn1 -- Controlled Current Source/LConn1 -- Voltage Measurement/LConn1
  A-/RConn1 -- Controlled Current Source/RConn1 -- Voltage Measurement/LConn2
  B+/RConn1 -- Voltage Measurement1/LConn1 -- Controlled Current Source1/LConn1
  B-/RConn1 -- Controlled Current Source1/RConn1 -- Voltage Measurement1/LConn2

== system DCE_motor6_V2/joint6/Motor1/Mechanical ==
  TL : Inport
  Te : Inport  Port=2
  1/J : Gain  Gain=1/(1e-5)
  B : Gain  Gain=1e-4
  Integrator : Integrator
  Integrator1 : Integrator
  Sum : Sum  Inputs=-+-
  w : Outport
  theta : Outport  Port=2
  wires:
  Te/1 -> Sum/2
  TL/1 -> Sum/1
  Sum/1 -> 1/J/1
  1/J/1 -> Integrator/1
  Integrator/1 -> B/1, w/1, Integrator1/1  "w"
  Integrator1/1 -> theta/1  "theta"
  B/1 -> Sum/3

== system DCE_motor6_V2/joint6/Motor2/Connector ==
  Ip : Inport
  Controlled Current Source : spsControlledCurrentSourceLib/Controlled Current Source  Initialize=on  Source_Type=AC  Amplitude=2  Phase=0  Frequency=0  Measurements=None
  Controlled Current Source1 : spsControlledCurrentSourceLib/Controlled Current Source  Initialize=on  Source_Type=AC  Amplitude=2  Phase=0  Frequency=0  Measurements=None
  Demux : Demux  Outputs=2
  Mux : Mux  Inputs=2
  Scope6 : Scope  NumInputPorts=2
      settings: ActiveDisplayYMinimum=-2.39364466431234  ActiveDisplayYMaximum=2.3993658884477673  DataLoggingVariableName=ScopeData5
  Voltage Measurement : spsVoltageMeasurementLib/Voltage Measurement  PhasorSimulation=off  OutputType=Complex  PSBequivalent=0
  Voltage Measurement1 : spsVoltageMeasurementLib/Voltage Measurement  PhasorSimulation=off  OutputType=Complex  PSBequivalent=0
  A+ : PMIOPort  Side=Left
  A- : PMIOPort  Port=2  Side=Left
  B+ : PMIOPort  Port=3  Side=Left
  B- : PMIOPort  Port=4  Side=Left
  Vp : Outport
  wires:
  Mux/1 -> Vp/1
  Ip/1 -> Demux/1
  Demux/1 -> Controlled Current Source/1
  Demux/2 -> Controlled Current Source1/1
  Voltage Measurement/1 -> Scope6/1, Mux/1  "Va"
  Voltage Measurement1/1 -> Scope6/2, Mux/2  "Vb"
  connections:
  A+/RConn1 -- Controlled Current Source/LConn1 -- Voltage Measurement/LConn1
  A-/RConn1 -- Controlled Current Source/RConn1 -- Voltage Measurement/LConn2
  B+/RConn1 -- Voltage Measurement1/LConn1 -- Controlled Current Source1/LConn1
  B-/RConn1 -- Controlled Current Source1/RConn1 -- Voltage Measurement1/LConn2

== system DCE_motor6_V2/joint6/Motor2/Mechanical ==
  TL : Inport
  Te : Inport  Port=2
  1/J : Gain  Gain=1/(1e-5)
  B : Gain  Gain=1e-4
  Integrator : Integrator
  Integrator1 : Integrator
  Sum : Sum  Inputs=-+-
  w : Outport
  theta : Outport  Port=2
  wires:
  Te/1 -> Sum/2
  TL/1 -> Sum/1
  Sum/1 -> 1/J/1
  1/J/1 -> Integrator/1
  Integrator/1 -> B/1, w/1, Integrator1/1  "w"
  Integrator1/1 -> theta/1  "theta"
  B/1 -> Sum/3

== system DCE_motor6_V2/powergui1/EquivalentModel1/Sources ==
  Mux : Mux  Inputs=[1 1]
  u : Outport  VectorParamsAs1DForOutWhenUnconnected=off
  wires:
  Mux/1 -> u/1
  [T52_4800_4466201355234] -> Mux/1
  [T68_6377_8151911135406] -> Mux/2

== system DCE_motor6_V2/powergui1/EquivalentModel1/Yout ==
  v,i : Inport
  Demux : Demux  Outputs=1
  tag scope: T64_6063_7583107454164=global
  wires:
  v,i/1 -> Demux/1
  Demux/1 -> [T64_6063_7583107454164]

== system DCE_motor6_V2/powergui1/EquivalentModel10/Sources ==
  Mux : Mux  Inputs=[1 1]
  u : Outport  VectorParamsAs1DForOutWhenUnconnected=off
  wires:
  Mux/1 -> u/1
  [T52_4803_4462221334465] -> Mux/1
  [T69_6428_8104491281436] -> Mux/2

== system DCE_motor6_V2/powergui1/EquivalentModel10/Yout ==
  v,i : Inport
  Demux : Demux  Outputs=1
  tag scope: T65_6114_7587207981716=global
  wires:
  v,i/1 -> Demux/1
  Demux/1 -> [T65_6114_7587207981716]

== system DCE_motor6_V2/powergui1/EquivalentModel11/Sources ==
  Mux : Mux  Inputs=[1 1]
  u : Outport  VectorParamsAs1DForOutWhenUnconnected=off
  wires:
  Mux/1 -> u/1
  [T52_4804_4462222168974] -> Mux/1
  [T68_6380_8144689156600] -> Mux/2

== system DCE_motor6_V2/powergui1/EquivalentModel11/Yout ==
  v,i : Inport
  Demux : Demux  Outputs=1
  tag scope: T64_6066_7575863512656=global
  wires:
  v,i/1 -> Demux/1
  Demux/1 -> [T64_6066_7575863512656]

== system DCE_motor6_V2/powergui1/EquivalentModel12/Sources ==
  Mux : Mux  Inputs=[1 1]
  u : Outport  VectorParamsAs1DForOutWhenUnconnected=off
  wires:
  Mux/1 -> u/1
  [T52_4805_4462365181946] -> Mux/1
  [T69_6429_8101879516219] -> Mux/2

== system DCE_motor6_V2/powergui1/EquivalentModel12/Yout ==
  v,i : Inport
  Demux : Demux  Outputs=1
  tag scope: T65_6115_7584604409678=global
  wires:
  v,i/1 -> Demux/1
  Demux/1 -> [T65_6115_7584604409678]

== system DCE_motor6_V2/powergui1/EquivalentModel13/Sources ==
  Mux : Mux  Inputs=[1 1]
  u : Outport  VectorParamsAs1DForOutWhenUnconnected=off
  wires:
  Mux/1 -> u/1
  [T52_4803_4460481445200] -> Mux/1
  [T68_6380_8145074705821] -> Mux/2

== system DCE_motor6_V2/powergui1/EquivalentModel13/Yout ==
  v,i : Inport
  Demux : Demux  Outputs=1
  tag scope: T64_6066_7576227462817=global
  wires:
  v,i/1 -> Demux/1
  Demux/1 -> [T64_6066_7576227462817]

== system DCE_motor6_V2/powergui1/EquivalentModel14/Sources ==
  Mux : Mux  Inputs=[1 1]
  u : Outport  VectorParamsAs1DForOutWhenUnconnected=off
  wires:
  Mux/1 -> u/1
  [T52_4804_4460338922847] -> Mux/1
  [T69_6429_8102260892805] -> Mux/2

== system DCE_motor6_V2/powergui1/EquivalentModel14/Yout ==
  v,i : Inport
  Demux : Demux  Outputs=1
  tag scope: T65_6115_7584964797990=global
  wires:
  v,i/1 -> Demux/1
  Demux/1 -> [T65_6115_7584964797990]

== system DCE_motor6_V2/powergui1/EquivalentModel15/Sources ==
  Mux : Mux  Inputs=[1 1]
  u : Outport  VectorParamsAs1DForOutWhenUnconnected=off
  wires:
  Mux/1 -> u/1
  [T52_4805_4460338578956] -> Mux/1
  [T68_6381_8142429380307] -> Mux/2

== system DCE_motor6_V2/powergui1/EquivalentModel15/Yout ==
  v,i : Inport
  Demux : Demux  Outputs=1
  tag scope: T64_6067_7573590378889=global
  wires:
  v,i/1 -> Demux/1
  Demux/1 -> [T64_6067_7573590378889]

== system DCE_motor6_V2/powergui1/EquivalentModel16/Sources ==
  Mux : Mux  Inputs=[1 1]
  u : Outport  VectorParamsAs1DForOutWhenUnconnected=off
  wires:
  Mux/1 -> u/1
  [T52_4806_4460480413526] -> Mux/1
  [T69_6430_8099648746360] -> Mux/2

== system DCE_motor6_V2/powergui1/EquivalentModel16/Yout ==
  v,i : Inport
  Demux : Demux  Outputs=1
  tag scope: T65_6116_7582360795971=global
  wires:
  v,i/1 -> Demux/1
  Demux/1 -> [T65_6116_7582360795971]

== system DCE_motor6_V2/powergui1/EquivalentModel17/Sources ==
  Mux : Mux  Inputs=[1 1]
  u : Outport  VectorParamsAs1DForOutWhenUnconnected=off
  wires:
  Mux/1 -> u/1
  [T52_4804_4458625615445] -> Mux/1
  [T68_6381_8142834748312] -> Mux/2

== system DCE_motor6_V2/powergui1/EquivalentModel17/Yout ==
  v,i : Inport
  Demux : Demux  Outputs=1
  tag scope: T64_6067_7573975412994=global
  wires:
  v,i/1 -> Demux/1
  Demux/1 -> [T64_6067_7573975412994]

== system DCE_motor6_V2/powergui1/EquivalentModel18/Sources ==
  Mux : Mux  Inputs=[1 1]
  u : Outport  VectorParamsAs1DForOutWhenUnconnected=off
  wires:
  Mux/1 -> u/1
  [T52_4805_4458481914691] -> Mux/1
  [T69_6430_8100049648811] -> Mux/2

== system DCE_motor6_V2/powergui1/EquivalentModel18/Yout ==
  v,i : Inport
  Demux : Demux  Outputs=1
  tag scope: T65_6116_7582741937034=global
  wires:
  v,i/1 -> Demux/1
  Demux/1 -> [T65_6116_7582741937034]

== system DCE_motor6_V2/powergui1/EquivalentModel19/Sources ==
  Mux : Mux  Inputs=[1 1]
  u : Outport  VectorParamsAs1DForOutWhenUnconnected=off
  wires:
  Mux/1 -> u/1
  [T52_4806_4458480392398] -> Mux/1
  [T68_6382_8140189030191] -> Mux/2

== system DCE_motor6_V2/powergui1/EquivalentModel19/Yout ==
  v,i : Inport
  Demux : Demux  Outputs=1
  tag scope: T64_6068_7571337885434=global
  wires:
  v,i/1 -> Demux/1
  Demux/1 -> [T64_6068_7571337885434]

== system DCE_motor6_V2/powergui1/EquivalentModel2/Sources ==
  Mux : Mux  Inputs=[1 1]
  u : Outport  VectorParamsAs1DForOutWhenUnconnected=off
  wires:
  Mux/1 -> u/1
  [T52_4801_4466062368084] -> Mux/1
  [T69_6426_8109009492613] -> Mux/2

== system DCE_motor6_V2/powergui1/EquivalentModel2/Yout ==
  v,i : Inport
  Demux : Demux  Outputs=1
  tag scope: T65_6112_7591755317476=global
  wires:
  v,i/1 -> Demux/1
  Demux/1 -> [T65_6112_7591755317476]

== system DCE_motor6_V2/powergui1/EquivalentModel20/Sources ==
  Mux : Mux  Inputs=[1 1]
  u : Outport  VectorParamsAs1DForOutWhenUnconnected=off
  wires:
  Mux/1 -> u/1
  [T52_4807_4458621048567] -> Mux/1
  [T69_6431_8097437121138] -> Mux/2

== system DCE_motor6_V2/powergui1/EquivalentModel20/Yout ==
  v,i : Inport
  Demux : Demux  Outputs=1
  tag scope: T65_6117_7580137505034=global
  wires:
  v,i/1 -> Demux/1
  Demux/1 -> [T65_6117_7580137505034]

== system DCE_motor6_V2/powergui1/EquivalentModel21/Sources ==
  Mux : Mux  Inputs=[1 1]
  u : Outport  VectorParamsAs1DForOutWhenUnconnected=off
  wires:
  Mux/1 -> u/1
  [T52_4805_4456795189152] -> Mux/1
  [T68_6382_8140614216980] -> Mux/2

== system DCE_motor6_V2/powergui1/EquivalentModel21/Yout ==
  v,i : Inport
  Demux : Demux  Outputs=1
  tag scope: T64_6068_7571744003482=global
  wires:
  v,i/1 -> Demux/1
  Demux/1 -> [T64_6068_7571744003482]
